simulink model "proyecto4_vss_orden3"  (Simulink 7.9)
settings: Solver=ode45  StartTime=0.0  StopTime=50  FixedStep=0.05  RelTol=1e-3
values from neighbouring files (symbols this model uses):
  KdL2 = 1    [graficacion_comp_orden.m]
  KdP2 = 18    [graficacion_comp_orden.m]
  KdX2 = 2    [graficacion_comp_orden.m]
  KuL2 = 1    [graficacion_comp_orden.m]
  KuP2 = 1    [graficacion_comp_orden.m]
  KuX2 = 1    [graficacion_comp_orden.m]
  LambdaL2 = 5    [graficacion_comp_orden.m]
  LambdaP2 = 1    [graficacion_comp_orden.m]
  LambdaX2 = 2    [graficacion_comp_orden.m]
libraries: simulink x3
settings Model: Creator=JuanPablo  LastModifiedBy=JuanPablo

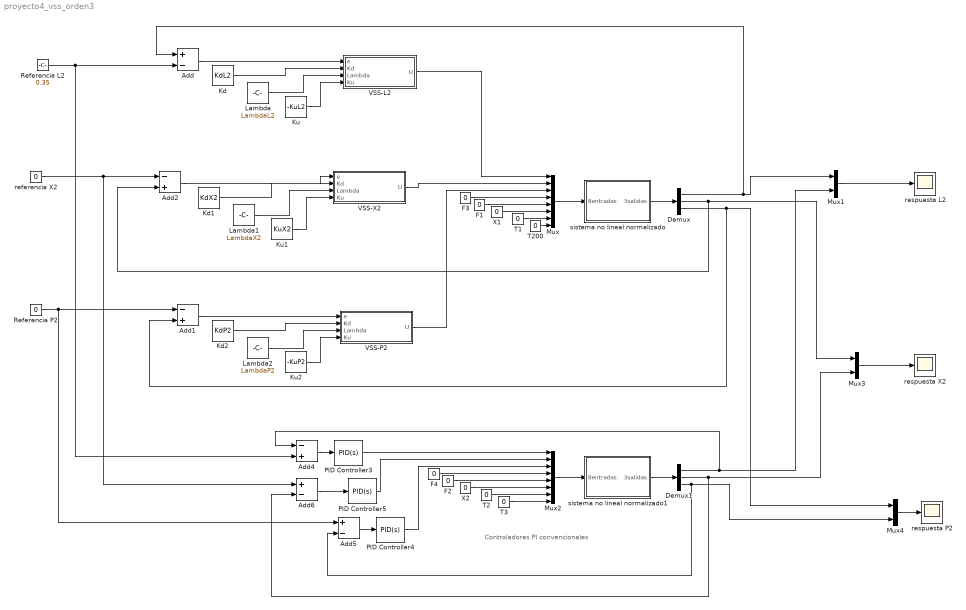
== system proyecto4_vss_orden3 ==
  note: Controladores PI convencionales
  Add : Sum  Inputs=+-
  Add1 : Sum  Inputs=-+
  Add2 : Sum  Inputs=-+
  Add4 : Sum  Inputs=-+
  Add5 : Sum  Inputs=+-
  Add6 : Sum  Inputs=+-
  Demux : Demux  Outputs=3
  Demux1 : Demux  Outputs=3
  F{1..4} (4 alike) : Constant  Value=0
  Kd : Constant  Value=KdL2
  Kd1 : Constant  Value=KdX2
  Kd2 : Constant  Value=KdP2
  Ku : Constant  Value=-KuL2
  Ku1 : Constant  Value=KuX2
  Ku2 : Constant  Value=-KuP2
  Lambda : Constant  Value=LambdaL2
  Lambda1 : Constant  Value=LambdaX2
  Lambda2 : Constant  Value=LambdaP2
  Mux : Mux  Inputs=8
  Mux1 : Mux  Inputs=2
  Mux2 : Mux  Inputs=8
  Mux3 : Mux  Inputs=2
  Mux4 : Mux  Inputs=2
  PID Controller3 : simulink/Continuous/PID Controller  Controller=PID  TimeDomain=Continuous-time  SampleTime=1  IntegratorMethod=Forward Euler  FilterMethod=Forward Euler  Form=Parallel  P=-7.5  I=0  D=0  N=100  InitialConditionSource=internal  InitialConditionForIntegrator=0  InitialConditionForFilter=0  ExternalReset=none  LimitOutput=off  UpperSaturationLimit=inf  LowerSaturationLimit=-inf  LinearizeAsGain=off  AntiWindupMode=none  Kb=1  TrackingMode=off  Kt=1  PParamMin=[]  PParamMax=[]  IParamMin=[]  IParamMax=[]  DParamMin=[]  DParamMax=[]  NParamMin=[]  NParamMax=[]  KbParamMin=[]  KbParamMax=[]  KtParamMin=[]  KtParamMax=[]  POutMin=[]  POutMax=[]  IOutMin=[]  IOutMax=[]  DOutMin=[]  DOutMax=[]  NOutMin=[]  NOutMax=[]  KbOutMin=[]  KbOutMax=[]  KtOutMin=[]  KtOutMax=[]  IntegratorOutMin=[]  IntegratorOutMax=[]  FilterOutMin=[]  FilterOutMax=[]  SumOutMin=[]  SumOutMax=[]  SumI1OutMin=[]  SumI1OutMax=[]  SumI2OutMin=[]  SumI2OutMax=[]  SumI3OutMin=[]  SumI3OutMax=[]  SumDOutMin=[]  SumDOutMax=[]  SaturationOutMin=[]  SaturationOutMax=[]  IntegratorContinuousStateAttributes=''  IntegratorStateMustResolveToSignalObject=off  IntegratorRTWStateStorageClass=Auto  FilterContinuousStateAttributes=''  FilterStateMustResolveToSignalObject=off  FilterRTWStateStorageClass=Auto
  PID Controller4 : simulink/Continuous/PID Controller  Controller=PID  TimeDomain=Continuous-time  SampleTime=1  IntegratorMethod=Forward Euler  FilterMethod=Forward Euler  Form=Parallel  P=-42.61364  I=-42.61364/10.989  D=0  N=100  InitialConditionSource=internal  InitialConditionForIntegrator=0  InitialConditionForFilter=0  ExternalReset=none  LimitOutput=off  UpperSaturationLimit=inf  LowerSaturationLimit=-inf  LinearizeAsGain=off  AntiWindupMode=none  Kb=1  TrackingMode=off  Kt=1  PParamMin=[]  PParamMax=[]  IParamMin=[]  IParamMax=[]  DParamMin=[]  DParamMax=[]  NParamMin=[]  NParamMax=[]  KbParamMin=[]  KbParamMax=[]  KtParamMin=[]  KtParamMax=[]  POutMin=[]  POutMax=[]  IOutMin=[]  IOutMax=[]  DOutMin=[]  DOutMax=[]  NOutMin=[]  NOutMax=[]  KbOutMin=[]  KbOutMax=[]  KtOutMin=[]  KtOutMax=[]  IntegratorOutMin=[]  IntegratorOutMax=[]  FilterOutMin=[]  FilterOutMax=[]  SumOutMin=[]  SumOutMax=[]  SumI1OutMin=[]  SumI1OutMax=[]  SumI2OutMin=[]  SumI2OutMax=[]  SumI3OutMin=[]  SumI3OutMax=[]  SumDOutMin=[]  SumDOutMax=[]  SaturationOutMin=[]  SaturationOutMax=[]  IntegratorContinuousStateAttributes=''  IntegratorStateMustResolveToSignalObject=off  IntegratorRTWStateStorageClass=Auto  FilterContinuousStateAttributes=''  FilterStateMustResolveToSignalObject=off  FilterRTWStateStorageClass=Auto
  PID Controller5 : simulink/Continuous/PID Controller  Controller=PID  TimeDomain=Continuous-time  SampleTime=1  IntegratorMethod=Forward Euler  FilterMethod=Forward Euler  Form=Parallel  P=3.70472  I=3.70472/2.664  D=0  N=100  InitialConditionSource=internal  InitialConditionForIntegrator=0  InitialConditionForFilter=0  ExternalReset=none  LimitOutput=off  UpperSaturationLimit=inf  LowerSaturationLimit=-inf  LinearizeAsGain=off  AntiWindupMode=none  Kb=1  TrackingMode=off  Kt=1  PParamMin=[]  PParamMax=[]  IParamMin=[]  IParamMax=[]  DParamMin=[]  DParamMax=[]  NParamMin=[]  NParamMax=[]  KbParamMin=[]  KbParamMax=[]  KtParamMin=[]  KtParamMax=[]  POutMin=[]  POutMax=[]  IOutMin=[]  IOutMax=[]  DOutMin=[]  DOutMax=[]  NOutMin=[]  NOutMax=[]  KbOutMin=[]  KbOutMax=[]  KtOutMin=[]  KtOutMax=[]  IntegratorOutMin=[]  IntegratorOutMax=[]  FilterOutMin=[]  FilterOutMax=[]  SumOutMin=[]  SumOutMax=[]  SumI1OutMin=[]  SumI1OutMax=[]  SumI2OutMin=[]  SumI2OutMax=[]  SumI3OutMin=[]  SumI3OutMax=[]  SumDOutMin=[]  SumDOutMax=[]  SaturationOutMin=[]  SaturationOutMax=[]  IntegratorContinuousStateAttributes=''  IntegratorStateMustResolveToSignalObject=off  IntegratorRTWStateStorageClass=Auto  FilterContinuousStateAttributes=''  FilterStateMustResolveToSignalObject=off  FilterRTWStateStorageClass=Auto
  Referencia L2 : Constant  Value=0.35
  Referencia P2 : Constant  Value=0
  T{1..3,200} (4 alike) : Constant  Value=0
  VSS-L2 : Subsystem  TreatAsAtomicUnit=on
  VSS-P2 : Subsystem  TreatAsAtomicUnit=on
  VSS-X2 : Subsystem  TreatAsAtomicUnit=on
  X1 : Constant  Value=0
  X2 : Constant  Value=0
  referencia X2 : Constant  Value=0
  respuesta L2 : Scope
      settings: TimeRange=50  YMin=-0.05  YMax=0.55  SaveName=closeloop_L2_orden3
  respuesta P2 : Scope
      settings: TimeRange=50  YMin=-0.02  YMax=0.02  SaveName=closeloop_P2_orden3
  respuesta X2 : Scope
      settings: TimeRange=50  YMin=-1.73472e-17  YMax=0.23  SaveName=closeloop_X2_orden3
  sistema no lineal normalizado : Subsystem  TreatAsAtomicUnit=on
  sistema no lineal normalizado1 : Subsystem  TreatAsAtomicUnit=on
  wires:
  Mux/1 -> sistema no lineal normalizado/1(8entradas)
  sistema no lineal normalizado/1(3salidas) -> Demux/1
  F3/1 -> Mux/4
  F1/1 -> Mux/5
  X1/1 -> Mux/6
  T1/1 -> Mux/7
  T200/1 -> Mux/8
  Demux/1 -> Add/1, Mux1/1
  Demux/2 -> Add2/2, Mux3/1
  Referencia L2/1 -> Add4/2, Add/2
  Referencia P2/1 -> Add5/1, Add1/1
  Demux/3 -> Add1/2, Mux4/1
  Mux2/1 -> sistema no lineal normalizado1/1(8entradas)
  sistema no lineal normalizado1/1(3salidas) -> Demux1/1
  F4/1 -> Mux2/4
  F2/1 -> Mux2/5
  X2/1 -> Mux2/6
  T2/1 -> Mux2/7
  T3/1 -> Mux2/8
  Demux1/1 -> Add4/1, Mux1/2
  Demux1/2 -> Add6/2, Mux3/2
  Add4/1 -> PID Controller3/1
  Add5/1 -> PID Controller4/1
  PID Controller4/1 -> Mux2/3
  Add6/1 -> PID Controller5/1
  PID Controller3/1 -> Mux2/1
  Demux1/3 -> Add5/2, Mux4/2
  PID Controller5/1 -> Mux2/2
  Mux1/1 -> respuesta L2/1
  Mux4/1 -> respuesta P2/1
  Mux3/1 -> respuesta X2/1
  referencia X2/1 -> Add2/1, Add6/1
  Add/1 -> VSS-L2/1(e)
  VSS-L2/1(U) -> Mux/1
  Kd/1 -> VSS-L2/2(Kd)
  Lambda/1 -> VSS-L2/3(Lambda)
  Ku/1 -> VSS-L2/4(Ku)
  VSS-X2/1(U) -> Mux/2
  VSS-P2/1(U) -> Mux/3
  Add2/1 -> VSS-X2/1(e)
  Kd1/1 -> VSS-X2/2(Kd)
  Lambda1/1 -> VSS-X2/3(Lambda)
  Ku1/1 -> VSS-X2/4(Ku)
  Add1/1 -> VSS-P2/1(e)
  Kd2/1 -> VSS-P2/2(Kd)
  Lambda2/1 -> VSS-P2/3(Lambda)
  Ku2/1 -> VSS-P2/4(Ku)

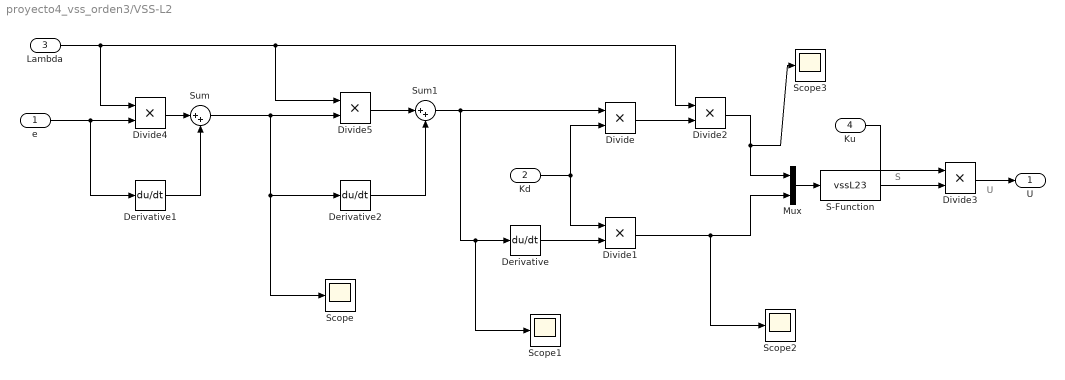
== system proyecto4_vss_orden3/VSS-L2 ==
  note: S
  note: U
  e : Inport
  Kd : Inport  Port=2
  Lambda : Inport  Port=3
  Ku : Inport  Port=4
  Derivative : Derivative
  Derivative1 : Derivative
  Derivative2 : Derivative
  Divide{,1..5} (6 alike) : Product  Inputs=**
  Mux : Mux  Inputs=2
  S-Function : S-Function  FunctionName=vssL23  EnableBusSupport=off
  Scope{,1..3} (4 alike) : Scope
      Scope settings: YMin=-4  YMax=0.5
      Scope1 settings: YMin=-125  YMax=100
      Scope2 settings: YMin=-175000  YMax=175000  SaveName=ScopeData2
      Scope3 settings: YMin=-5000  YMax=5000  SaveName=ScopeData3
  Sum : Sum  Inputs=|++
  Sum1 : Sum  Inputs=|++
  U : Outport
  wires:
  Derivative/1 -> Divide1/2
  Kd/1 -> Divide/2, Divide1/1
  Divide/1 -> Divide2/2
  Lambda/1 -> Divide4/1, Divide2/1, Divide5/1
  Divide1/1 -> Mux/2, Scope2/1
  Divide2/1 -> Mux/1, Scope3/1
  Mux/1 -> S-Function/1
  S-Function/1 -> Divide3/2
  Divide3/1 -> U/1
  Ku/1 -> Divide3/1
  e/1 -> Divide4/2, Derivative1/1
  Divide4/1 -> Sum/1
  Derivative1/1 -> Sum/2
  Divide5/1 -> Sum1/1
  Derivative2/1 -> Sum1/2
  Sum/1 -> Divide5/2, Derivative2/1, Scope/1
  Sum1/1 -> Divide/1, Derivative/1, Scope1/1

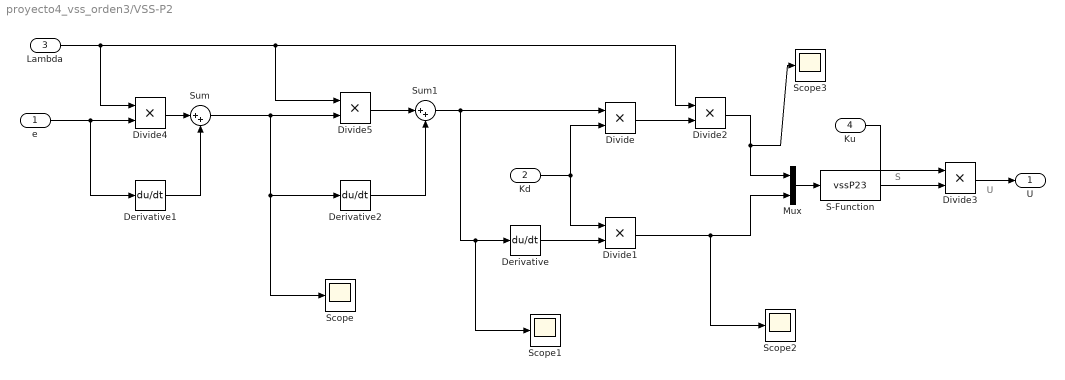
== system proyecto4_vss_orden3/VSS-P2 ==
  note: S
  note: U
  e : Inport
  Kd : Inport  Port=2
  Lambda : Inport  Port=3
  Ku : Inport  Port=4
  Derivative : Derivative
  Derivative1 : Derivative
  Derivative2 : Derivative
  Divide{,1..5} (6 alike) : Product  Inputs=**
  Mux : Mux  Inputs=2
  S-Function : S-Function  FunctionName=vssP23  EnableBusSupport=off
  Scope{,1..3} (4 alike) : Scope
      Scope settings: YMin=-4  YMax=0.5
      Scope1 settings: YMin=-125  YMax=100
      Scope2 settings: YMin=-200000  YMax=225000  SaveName=ScopeData2
      Scope3 settings: YMin=-1250  YMax=1250  SaveName=ScopeData3
  Sum : Sum  Inputs=|++
  Sum1 : Sum  Inputs=|++
  U : Outport
  wires:
  Derivative/1 -> Divide1/2
  Kd/1 -> Divide/2, Divide1/1
  Divide/1 -> Divide2/2
  Lambda/1 -> Divide4/1, Divide2/1, Divide5/1
  Divide1/1 -> Mux/2, Scope2/1
  Divide2/1 -> Mux/1, Scope3/1
  Mux/1 -> S-Function/1
  S-Function/1 -> Divide3/2
  Divide3/1 -> U/1
  Ku/1 -> Divide3/1
  e/1 -> Divide4/2, Derivative1/1
  Divide4/1 -> Sum/1
  Derivative1/1 -> Sum/2
  Divide5/1 -> Sum1/1
  Derivative2/1 -> Sum1/2
  Sum/1 -> Divide5/2, Derivative2/1, Scope/1
  Sum1/1 -> Divide/1, Derivative/1, Scope1/1

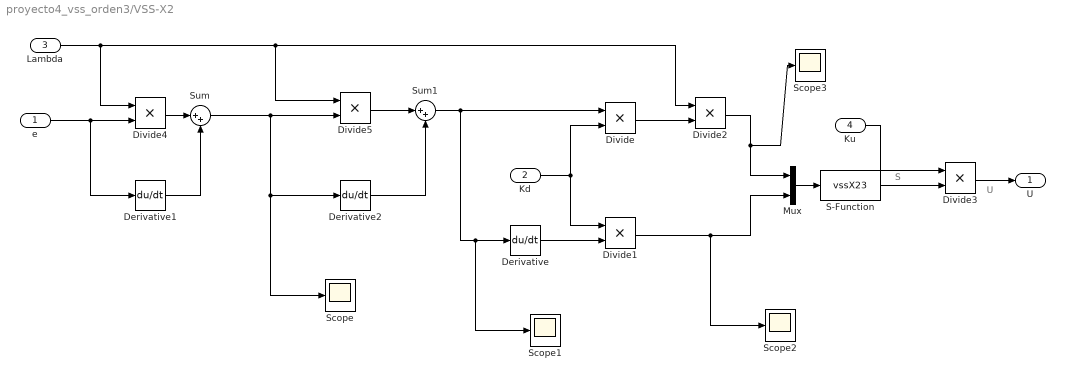
== system proyecto4_vss_orden3/VSS-X2 ==
  note: S
  note: U
  e : Inport
  Kd : Inport  Port=2
  Lambda : Inport  Port=3
  Ku : Inport  Port=4
  Derivative : Derivative
  Derivative1 : Derivative
  Derivative2 : Derivative
  Divide{,1..5} (6 alike) : Product  Inputs=**
  Mux : Mux  Inputs=2
  S-Function : S-Function  FunctionName=vssX23  EnableBusSupport=off
  Scope{,1..3} (4 alike) : Scope
      Scope settings: YMin=-4  YMax=0.5
      Scope1 settings: YMin=-125  YMax=100
      Scope2 settings: YMin=-2500  YMax=4000  SaveName=ScopeData2
      Scope3 settings: YMin=-175  YMax=100  SaveName=ScopeData3
  Sum : Sum  Inputs=|++
  Sum1 : Sum  Inputs=|++
  U : Outport
  wires:
  Derivative/1 -> Divide1/2
  Kd/1 -> Divide/2, Divide1/1
  Divide/1 -> Divide2/2
  Lambda/1 -> Divide4/1, Divide2/1, Divide5/1
  Divide1/1 -> Mux/2, Scope2/1
  Divide2/1 -> Mux/1, Scope3/1
  Mux/1 -> S-Function/1
  S-Function/1 -> Divide3/2
  Divide3/1 -> U/1
  Ku/1 -> Divide3/1
  e/1 -> Divide4/2, Derivative1/1
  Divide4/1 -> Sum/1
  Derivative1/1 -> Sum/2
  Divide5/1 -> Sum1/1
  Derivative2/1 -> Sum1/2
  Sum/1 -> Divide5/2, Derivative2/1, Scope/1
  Sum1/1 -> Divide/1, Derivative/1, Scope1/1

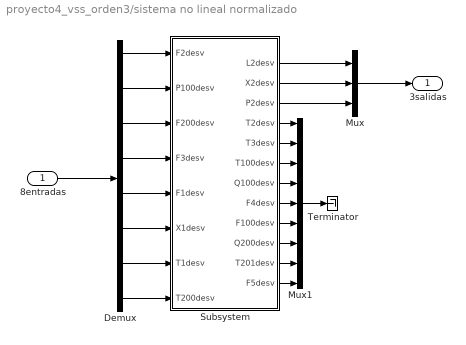
== system proyecto4_vss_orden3/sistema no lineal normalizado ==
  8entradas : Inport
  Demux : Demux  Outputs=8
  Mux : Mux  Inputs=3
  Mux1 : Mux  Inputs=9
  Subsystem : Subsystem
  Terminator : Terminator
  3salidas : Outport
  wires:
  8entradas/1 -> Demux/1
  Demux/1 -> Subsystem/1(F2desv)
  Demux/2 -> Subsystem/2(P100desv)
  Demux/3 -> Subsystem/3(F200desv)
  Demux/4 -> Subsystem/4(F3desv)
  Demux/5 -> Subsystem/5(F1desv)
  Demux/6 -> Subsystem/6(X1desv)
  Demux/7 -> Subsystem/7(T1desv)
  Demux/8 -> Subsystem/8(T200desv)
  Subsystem/1(L2desv) -> Mux/1
  Subsystem/2(X2desv) -> Mux/2
  Subsystem/3(P2desv) -> Mux/3
  Mux/1 -> 3salidas/1
  Subsystem/4(T2desv) -> Mux1/1
  Subsystem/5(T3desv) -> Mux1/2
  Subsystem/6(T100desv) -> Mux1/3
  Subsystem/7(Q100desv) -> Mux1/4
  Subsystem/8(F4desv) -> Mux1/5
  Subsystem/9(F100desv) -> Mux1/6
  Subsystem/10(Q200desv) -> Mux1/7
  Subsystem/11(T201desv) -> Mux1/8
  Subsystem/12(F5desv) -> Mux1/9
  Mux1/1 -> Terminator/1

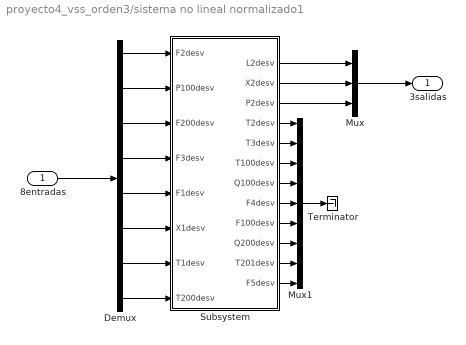
== system proyecto4_vss_orden3/sistema no lineal normalizado1 ==
  8entradas : Inport
  Demux : Demux  Outputs=8
  Mux : Mux  Inputs=3
  Mux1 : Mux  Inputs=9
  Subsystem : Subsystem
  Terminator : Terminator
  3salidas : Outport
  wires:
  8entradas/1 -> Demux/1
  Demux/1 -> Subsystem/1(F2desv)
  Demux/2 -> Subsystem/2(P100desv)
  Demux/3 -> Subsystem/3(F200desv)
  Demux/4 -> Subsystem/4(F3desv)
  Demux/5 -> Subsystem/5(F1desv)
  Demux/6 -> Subsystem/6(X1desv)
  Demux/7 -> Subsystem/7(T1desv)
  Demux/8 -> Subsystem/8(T200desv)
  Subsystem/1(L2desv) -> Mux/1
  Subsystem/2(X2desv) -> Mux/2
  Subsystem/3(P2desv) -> Mux/3
  Mux/1 -> 3salidas/1
  Subsystem/4(T2desv) -> Mux1/1
  Subsystem/5(T3desv) -> Mux1/2
  Subsystem/6(T100desv) -> Mux1/3
  Subsystem/7(Q100desv) -> Mux1/4
  Subsystem/8(F4desv) -> Mux1/5
  Subsystem/9(F100desv) -> Mux1/6
  Subsystem/10(Q200desv) -> Mux1/7
  Subsystem/11(T201desv) -> Mux1/8
  Subsystem/12(F5desv) -> Mux1/9
  Mux1/1 -> Terminator/1

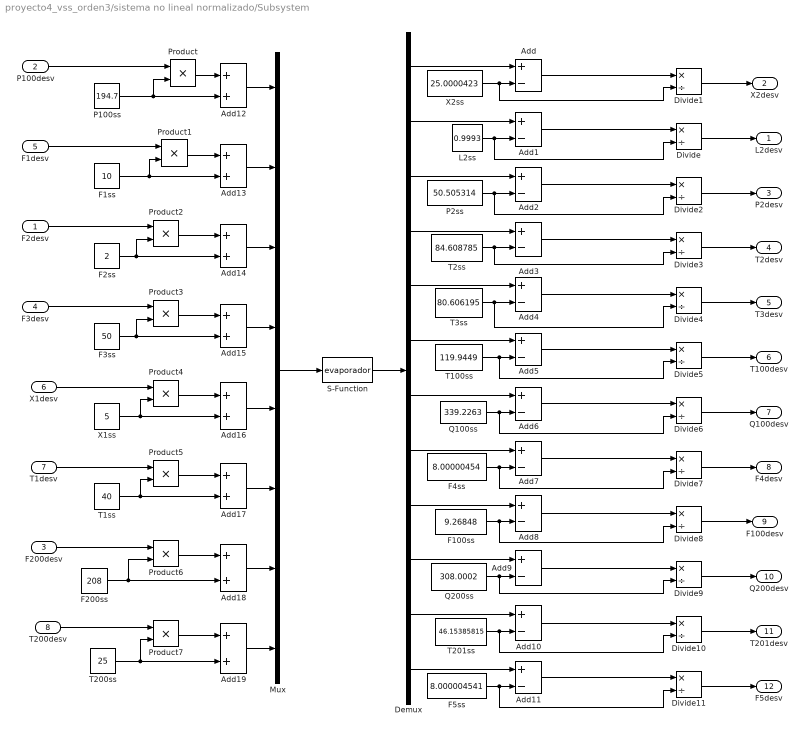
== system proyecto4_vss_orden3/sistema no lineal normalizado/Subsystem ==
  F2desv : Inport
  P100desv : Inport  Port=2
  F200desv : Inport  Port=3
  F3desv : Inport  Port=4
  F1desv : Inport  Port=5
  X1desv : Inport  Port=6
  T1desv : Inport  Port=7
  T200desv : Inport  Port=8
  Add{,1..11} (12 alike) : Sum  Inputs=+-
  Add{12..19} (8 alike) : Sum
  Demux : Demux  Outputs=12
  Divide{,1..11} (12 alike) : Product  Inputs=*/
  F100ss : Constant  Value=9.26848
  F1ss : Constant  Value=10
  F200ss : Constant  Value=208
  F2ss : Constant  Value=2
  F3ss : Constant  Value=50
  F4ss : Constant  Value=8.00000454
  F5ss : Constant  Value=8.000004541
  L2ss : Constant  Value=0.9993
  Mux : Mux  Inputs=8
  P100ss : Constant  Value=194.7
  P2ss : Constant  Value=50.505314
  Product{,1..7} (8 alike) : Product  RndMeth=Zero
  Q100ss : Constant  Value=339.2263
  Q200ss : Constant  Value=308.0002
  S-Function : S-Function  FunctionName=evaporador  EnableBusSupport=off
  T100ss : Constant  Value=119.9449
  T1ss : Constant  Value=40
  T200ss : Constant  Value=25
  T201ss : Constant  Value=46.15385815
  T2ss : Constant  Value=84.608785
  T3ss : Constant  Value=80.606195
  X1ss : Constant  Value=5
  X2ss : Constant  Value=25.0000423
  L2desv : Outport
  X2desv : Outport  Port=2
  P2desv : Outport  Port=3
  T2desv : Outport  Port=4
  T3desv : Outport  Port=5
  T100desv : Outport  Port=6
  Q100desv : Outport  Port=7
  F4desv : Outport  Port=8
  F100desv : Outport  Port=9
  Q200desv : Outport  Port=10
  T201desv : Outport  Port=11
  F5desv : Outport  Port=12
  wires:
  Mux/1 -> S-Function/1
  S-Function/1 -> Demux/1
  Demux/1 -> Add/1
  X2ss/1 -> Add/2, Divide1/2
  Demux/2 -> Add1/1
  L2ss/1 -> Add1/2, Divide/2
  Demux/3 -> Add2/1
  P2ss/1 -> Add2/2, Divide2/2
  Demux/4 -> Add3/1
  T2ss/1 -> Add3/2, Divide3/2
  Demux/5 -> Add4/1
  T3ss/1 -> Add4/2, Divide4/2
  Demux/6 -> Add5/1
  T100ss/1 -> Add5/2, Divide5/2
  Demux/7 -> Add6/1
  Q100ss/1 -> Add6/2, Divide6/2
  Demux/8 -> Add7/1
  F4ss/1 -> Add7/2, Divide7/2
  Demux/9 -> Add8/1
  F100ss/1 -> Add8/2, Divide8/2
  Demux/10 -> Add9/1
  Q200ss/1 -> Add9/2, Divide9/2
  Demux/11 -> Add10/1
  T201ss/1 -> Add10/2, Divide10/2
  Demux/12 -> Add11/1
  F5ss/1 -> Add11/2, Divide11/2
  P100ss/1 -> Add12/2, Product/2
  Add12/1 -> Mux/1
  F1ss/1 -> Add13/2, Product1/2
  Add13/1 -> Mux/2
  F2ss/1 -> Add14/2, Product2/2
  Add14/1 -> Mux/3
  F3ss/1 -> Add15/2, Product3/2
  Add15/1 -> Mux/4
  X1ss/1 -> Add16/2, Product4/2
  Add16/1 -> Mux/5
  T1ss/1 -> Add17/2, Product5/2
  Add17/1 -> Mux/6
  F200ss/1 -> Add18/2, Product6/2
  Add18/1 -> Mux/7
  T200ss/1 -> Add19/2, Product7/2
  Add19/1 -> Mux/8
  Product/1 -> Add12/1
  P100desv/1 -> Product/1
  Add1/1 -> Divide/1
  Divide/1 -> L2desv/1
  Product1/1 -> Add13/1
  F1desv/1 -> Product1/1
  Product2/1 -> Add14/1
  F2desv/1 -> Product2/1
  Product3/1 -> Add15/1
  F3desv/1 -> Product3/1
  X1desv/1 -> Product4/1
  Product4/1 -> Add16/1
  Product5/1 -> Add17/1
  T1desv/1 -> Product5/1
  Product6/1 -> Add18/1
  F200desv/1 -> Product6/1
  T200desv/1 -> Product7/1
  Product7/1 -> Add19/1
  Divide1/1 -> X2desv/1
  Add/1 -> Divide1/1
  Divide2/1 -> P2desv/1
  Add2/1 -> Divide2/1
  Divide3/1 -> T2desv/1
  Add3/1 -> Divide3/1
  Add4/1 -> Divide4/1
  Divide4/1 -> T3desv/1
  Divide5/1 -> T100desv/1
  Add5/1 -> Divide5/1
  Divide6/1 -> Q100desv/1
  Add6/1 -> Divide6/1
  Divide7/1 -> F4desv/1
  Add7/1 -> Divide7/1
  Divide8/1 -> F100desv/1
  Add8/1 -> Divide8/1
  Divide9/1 -> Q200desv/1
  Add9/1 -> Divide9/1
  Divide10/1 -> T201desv/1
  Add10/1 -> Divide10/1
  Divide11/1 -> F5desv/1
  Add11/1 -> Divide11/1

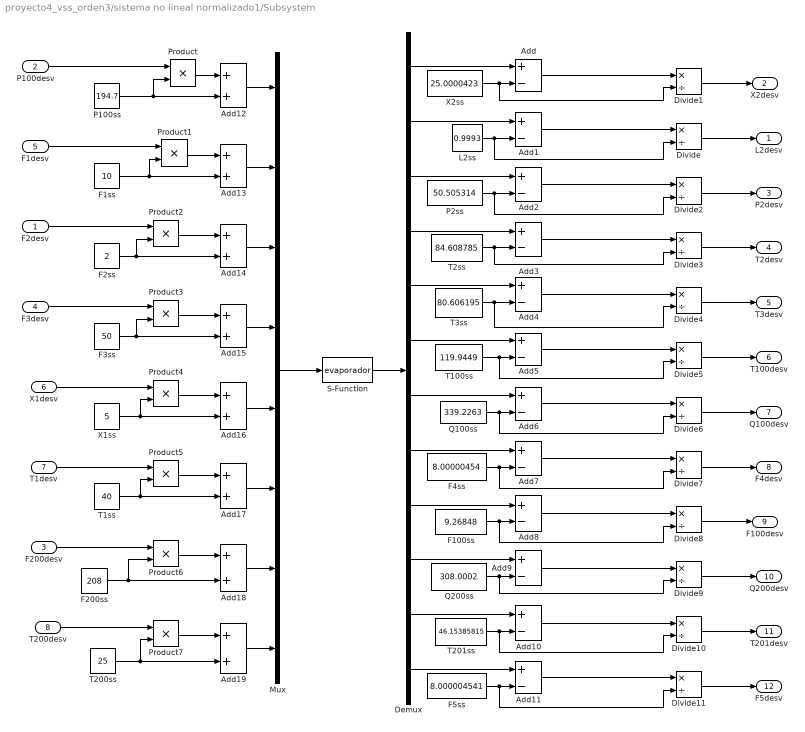
== system proyecto4_vss_orden3/sistema no lineal normalizado1/Subsystem ==
  F2desv : Inport
  P100desv : Inport  Port=2
  F200desv : Inport  Port=3
  F3desv : Inport  Port=4
  F1desv : Inport  Port=5
  X1desv : Inport  Port=6
  T1desv : Inport  Port=7
  T200desv : Inport  Port=8
  Add{,1..11} (12 alike) : Sum  Inputs=+-
  Add{12..19} (8 alike) : Sum
  Demux : Demux  Outputs=12
  Divide{,1..11} (12 alike) : Product  Inputs=*/
  F100ss : Constant  Value=9.26848
  F1ss : Constant  Value=10
  F200ss : Constant  Value=208
  F2ss : Constant  Value=2
  F3ss : Constant  Value=50
  F4ss : Constant  Value=8.00000454
  F5ss : Constant  Value=8.000004541
  L2ss : Constant  Value=0.9993
  Mux : Mux  Inputs=8
  P100ss : Constant  Value=194.7
  P2ss : Constant  Value=50.505314
  Product{,1..7} (8 alike) : Product  RndMeth=Zero
  Q100ss : Constant  Value=339.2263
  Q200ss : Constant  Value=308.0002
  S-Function : S-Function  FunctionName=evaporador  EnableBusSupport=off
  T100ss : Constant  Value=119.9449
  T1ss : Constant  Value=40
  T200ss : Constant  Value=25
  T201ss : Constant  Value=46.15385815
  T2ss : Constant  Value=84.608785
  T3ss : Constant  Value=80.606195
  X1ss : Constant  Value=5
  X2ss : Constant  Value=25.0000423
  L2desv : Outport
  X2desv : Outport  Port=2
  P2desv : Outport  Port=3
  T2desv : Outport  Port=4
  T3desv : Outport  Port=5
  T100desv : Outport  Port=6
  Q100desv : Outport  Port=7
  F4desv : Outport  Port=8
  F100desv : Outport  Port=9
  Q200desv : Outport  Port=10
  T201desv : Outport  Port=11
  F5desv : Outport  Port=12
  wires:
  Mux/1 -> S-Function/1
  S-Function/1 -> Demux/1
  Demux/1 -> Add/1
  X2ss/1 -> Add/2, Divide1/2
  Demux/2 -> Add1/1
  L2ss/1 -> Add1/2, Divide/2
  Demux/3 -> Add2/1
  P2ss/1 -> Add2/2, Divide2/2
  Demux/4 -> Add3/1
  T2ss/1 -> Add3/2, Divide3/2
  Demux/5 -> Add4/1
  T3ss/1 -> Add4/2, Divide4/2
  Demux/6 -> Add5/1
  T100ss/1 -> Add5/2, Divide5/2
  Demux/7 -> Add6/1
  Q100ss/1 -> Add6/2, Divide6/2
  Demux/8 -> Add7/1
  F4ss/1 -> Add7/2, Divide7/2
  Demux/9 -> Add8/1
  F100ss/1 -> Add8/2, Divide8/2
  Demux/10 -> Add9/1
  Q200ss/1 -> Add9/2, Divide9/2
  Demux/11 -> Add10/1
  T201ss/1 -> Add10/2, Divide10/2
  Demux/12 -> Add11/1
  F5ss/1 -> Add11/2, Divide11/2
  P100ss/1 -> Add12/2, Product/2
  Add12/1 -> Mux/1
  F1ss/1 -> Add13/2, Product1/2
  Add13/1 -> Mux/2
  F2ss/1 -> Add14/2, Product2/2
  Add14/1 -> Mux/3
  F3ss/1 -> Add15/2, Product3/2
  Add15/1 -> Mux/4
  X1ss/1 -> Add16/2, Product4/2
  Add16/1 -> Mux/5
  T1ss/1 -> Add17/2, Product5/2
  Add17/1 -> Mux/6
  F200ss/1 -> Add18/2, Product6/2
  Add18/1 -> Mux/7
  T200ss/1 -> Add19/2, Product7/2
  Add19/1 -> Mux/8
  Product/1 -> Add12/1
  P100desv/1 -> Product/1
  Add1/1 -> Divide/1
  Divide/1 -> L2desv/1
  Product1/1 -> Add13/1
  F1desv/1 -> Product1/1
  Product2/1 -> Add14/1
  F2desv/1 -> Product2/1
  Product3/1 -> Add15/1
  F3desv/1 -> Product3/1
  X1desv/1 -> Product4/1
  Product4/1 -> Add16/1
  Product5/1 -> Add17/1
  T1desv/1 -> Product5/1
  Product6/1 -> Add18/1
  F200desv/1 -> Product6/1
  T200desv/1 -> Product7/1
  Product7/1 -> Add19/1
  Divide1/1 -> X2desv/1
  Add/1 -> Divide1/1
  Divide2/1 -> P2desv/1
  Add2/1 -> Divide2/1
  Divide3/1 -> T2desv/1
  Add3/1 -> Divide3/1
  Add4/1 -> Divide4/1
  Divide4/1 -> T3desv/1
  Divide5/1 -> T100desv/1
  Add5/1 -> Divide5/1
  Divide6/1 -> Q100desv/1
  Add6/1 -> Divide6/1
  Divide7/1 -> F4desv/1
  Add7/1 -> Divide7/1
  Divide8/1 -> F100desv/1
  Add8/1 -> Divide8/1
  Divide9/1 -> Q200desv/1
  Add9/1 -> Divide9/1
  Divide10/1 -> T201desv/1
  Add10/1 -> Divide10/1
  Divide11/1 -> F5desv/1
  Add11/1 -> Divide11/1
